simulink model "LoopStructure_Designmodel"  (R2020b)
settings: Solver=VariableStepAuto  StartTime=0.0  StopTime=10.0  RelTol=1e-3
settings Model: Creator=Administrator  LastModifiedBy=Administrator

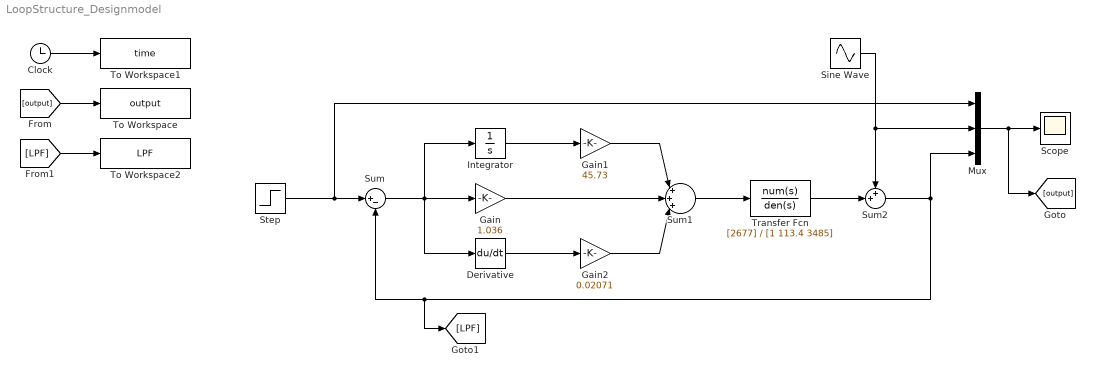
== system LoopStructure_Designmodel ==
  Clock : Clock
  Derivative : Derivative
  Gain : Gain  Gain=1.036
  Gain1 : Gain  Tag=z  Gain=45.73
  Gain2 : Gain  Gain=0.02071
  Integrator : Integrator
  Mux : Mux  Inputs=3
  Scope : Scope
  Sine Wave : Sin  Frequency=5  SampleTime=0
  Step : Step  After=0  SampleTime=0
  Sum : Sum  Inputs=|+-
  Sum1 : Sum  Inputs=|+++|
  Sum2 : Sum  Inputs=++|
  To Workspace : ToWorkspace  VariableName=output  SampleTime=-1
  To Workspace1 : ToWorkspace  VariableName=time  SampleTime=-1
  To Workspace2 : ToWorkspace  VariableName=LPF  SaveFormat=Timeseries  SampleTime=-1
  Transfer Fcn : TransferFcn  Numerator=[2677]  Denominator=[1 113.4 3485]
  wires:
  Step/1 -> Mux/1, Sum/1
  Integrator/1 -> Gain1/1
  Gain2/1 -> Sum1/3
  Gain/1 -> Sum1/2
  Gain1/1 -> Sum1/1
  Derivative/1 -> Gain2/1
  Sum/1 -> Derivative/1, Gain/1, Integrator/1
  Sum1/1 -> Transfer Fcn/1
  Transfer Fcn/1 -> Sum2/2
  Sum2/1 -> Mux/3, [LPF], Sum/2
  Sine Wave/1 -> Sum2/1, Mux/2
  Mux/1 -> [output], Scope/1
  Clock/1 -> To Workspace1/1
  [output] -> To Workspace/1
  [LPF] -> To Workspace2/1
